simulink model "scheme"  (R2021b)
settings: Solver=FixedStepAuto  StartTime=0.0  StopTime=0.7  FixedStep=1e-4  RelTol=1e-3
undefined symbols (not defined in the file): k1, k2, k3
libraries: fuzblock x2
settings Model: Creator=vkad  LastModifiedBy=vkad

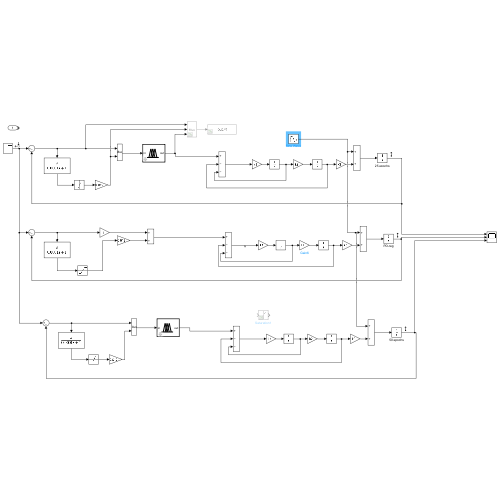
[thumbnail: Simulink's stored preview of the top-level diagram]
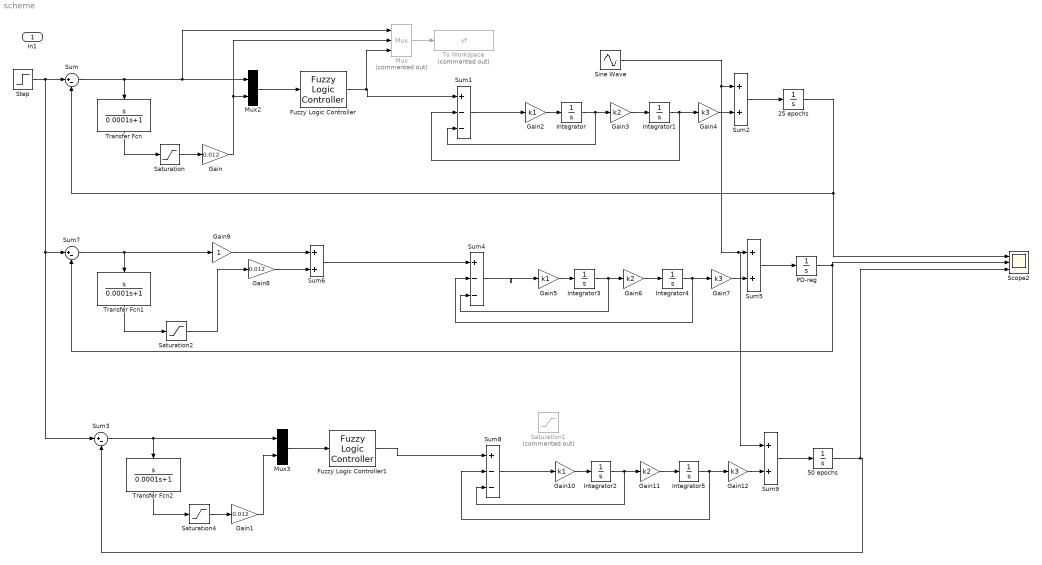
== system scheme ==
  In1 : Inport
  25 epochs : Integrator
  50 epochs : Integrator
  Fuzzy Logic Controller : fuzblock/Fuzzy Logic  Controller  FIS=sugeno_25  OutputSampleNumber=101  DataType=double  FuzzifiedInputs=off  RuleFiringStrengths=off  RuleOutputs=off  AggregatedOutputs=off  SimulateUsing=Interpreted execution  OutOfRangeInputValueMessage=warning  NoRuleFiredMessage=warning  EmptyOutputFuzzySetMessage=warning
  Fuzzy Logic Controller1 : fuzblock/Fuzzy Logic  Controller  FIS=sugeno_50  OutputSampleNumber=101  DataType=double  FuzzifiedInputs=off  RuleFiringStrengths=off  RuleOutputs=off  AggregatedOutputs=off  SimulateUsing=Interpreted execution  OutOfRangeInputValueMessage=warning  NoRuleFiredMessage=warning  EmptyOutputFuzzySetMessage=warning
  Gain : Gain  Gain=0.012
  Gain1 : Gain  Gain=0.012
  Gain10 : Gain  Gain=k1
  Gain11 : Gain  Gain=k2
  Gain12 : Gain  Gain=k3
  Gain2 : Gain  Gain=k1
  Gain3 : Gain  Gain=k2
  Gain4 : Gain  Gain=k3
  Gain5 : Gain  Gain=k1
  Gain6 : Gain  Gain=k2
  Gain7 : Gain  Gain=k3
  Gain8 : Gain  Gain=0.012
  Gain9 : Gain
  Integrator{,1..5} (6 alike) : Integrator
  Mux : Mux  Commented=on  Inputs=3
  Mux2 : Mux  Inputs=2
  Mux3 : Mux  Inputs=2
  PD-reg : Integrator
  Saturation : Saturate
  Saturation1 : Saturate  Commented=on  UpperLimit=0.15  LowerLimit=-0.15  LinearizeAsGain=off
  Saturation2 : Saturate
  Saturation4 : Saturate
  Scope2 : Scope  NumInputPorts=3
  Sine Wave : Sin  Amplitude=20  Frequency=80  Phase=pi/3  SampleTime=0
  Step : Step  Time=0  SampleTime=0
  Sum : Sum  Inputs=|+-
  Sum1 : Sum  Inputs=+--
  Sum{2,5..6,9} (4 alike) : Sum
  Sum3 : Sum  Inputs=|+-
  Sum4 : Sum  Inputs=+--
  Sum7 : Sum  Inputs=|+-
  Sum8 : Sum  Inputs=+--
  To Workspace : ToWorkspace  Commented=on  VariableName=vf  SaveFormat=Timeseries  SampleTime=-1
  Transfer Fcn : TransferFcn  Numerator=[1 0]  Denominator=[0.0001 1]
  Transfer Fcn1 : TransferFcn  Numerator=[1 0]  Denominator=[0.0001 1]
  Transfer Fcn2 : TransferFcn  Numerator=[1 0]  Denominator=[0.0001 1]
  wires:
  Sum/1 -> Mux/1, Mux2/1, Transfer Fcn/1
  Transfer Fcn/1 -> Saturation/1
  Saturation/1 -> Gain/1
  Gain/1 -> Mux2/2, Mux/2
  Mux2/1 -> Fuzzy Logic Controller/1
  Fuzzy Logic Controller/1 -> Sum1/1, Mux/3
  Gain2/1 -> Integrator/1
  Gain3/1 -> Integrator1/1
  Integrator/1 -> Sum1/3, Gain3/1
  Integrator1/1 -> Sum1/2, Gain4/1
  25 epochs/1 -> Sum/2, Scope2/1
  Gain4/1 -> Sum2/2
  Sum2/1 -> 25 epochs/1
  Mux/1 -> To Workspace/1
  Sum5/1 -> PD-reg/1
  Gain7/1 -> Sum5/2
  PD-reg/1 -> Scope2/2, Sum7/2
  Integrator4/1 -> Sum4/2, Gain7/1
  Integrator3/1 -> Sum4/3, Gain6/1
  Gain6/1 -> Integrator4/1
  Gain5/1 -> Integrator3/1
  Sum6/1 -> Sum4/1
  Gain9/1 -> Sum6/1
  Gain8/1 -> Sum6/2
  Saturation2/1 -> Gain8/1
  Transfer Fcn1/1 -> Saturation2/1
  Sum7/1 -> Transfer Fcn1/1, Gain9/1
  Transfer Fcn2/1 -> Saturation4/1
  Step/1 -> Sum3/1, Sum7/1, Sum/1
  Fuzzy Logic Controller1/1 -> Sum8/1
  Gain12/1 -> Sum9/2
  Sine Wave/1 -> Sum9/1, Sum5/1, Sum2/1
  Sum9/1 -> 50 epochs/1
  Gain11/1 -> Integrator5/1
  Gain1/1 -> Mux3/2
  Integrator2/1 -> Sum8/3, Gain11/1
  Gain10/1 -> Integrator2/1
  Sum3/1 -> Mux3/1, Transfer Fcn2/1
  Saturation4/1 -> Gain1/1
  Integrator5/1 -> Sum8/2, Gain12/1
  50 epochs/1 -> Scope2/3, Sum3/2
  Mux3/1 -> Fuzzy Logic Controller1/1
  Sum4/1 -> Gain5/1
  Sum1/1 -> Gain2/1
  Sum8/1 -> Gain10/1
